simulink model "w31_v6"  (Simulink 7.9)
settings: Solver=FixedStepDiscrete  StartTime=0.0  StopTime=inf  FixedStep=0.01  RelTol=1e-3
undefined symbols (not defined in the file): DiscIntNeverNeededParam, magnitude
libraries: canmsglib x24, cansrvlib x22, simulink x12, iohwablib x5, legionoslib x3, ccpsrvlib x2, memsrvlib x1, tgttoollib x1, udssrvlib x1, wdgmlib x1
(part 1 of 5)
settings Model: Creator=jjlong  LastModifiedBy=申棋仁
settings DataIOCC: SaveOutput=off  SignalLogging=off  DSMLogging=off  SaveTime=off
settings OptimizationCC: InlineParams=on  ZeroExternalMemoryAtStartup=off  NoFixptDivByZeroProtection=on  EfficientFloat2IntCast=on  OptimizeModelRefInitCode=on  LifeSpan=1
settings DebuggingCC: ParameterOverflowMsg=none  ParameterPrecisionLossMsg=none  FrameProcessingCompatibilityMsg=error  StrictBusMsg=Warning
settings HardwareCC: ProdBitPerChar=16  ProdBitPerInt=16  ProdBitPerPointer=16  ProdLargestAtomicInteger=Integer  ProdIntDivRoundTo=Zero  ProdEndianess=LittleEndian  ProdWordSize=16  ProdHWDeviceType=Texas Instruments->C2000
settings RTWCC: SystemTargetFile=ez_ert_rtw.tlc  TemplateMakefile=ez_ert_rtw.tmf  Description=ControlKernel(tm) Rapid Prototyping  ProcessScript=ez_ert_rtw_make_rtw_hook
settings CodeAppCC: IgnoreCustomStorageClasses=off
settings STFCustomTargetCC: CodeReplacementLibrary=C89/C90 (ANSI)  CompOptLevelCompliant=on  IncludeMdlTerminateFcn=off  CombineOutputUpdateFcns=on  ERTFirstTimeCompliant=on  ERTCustomFileBanners=on  SupportNonFinite=off  SupportContinuousTime=off  SupportNonInlinedSFcns=off  GRTInterface=off  SystemTargetFile=ez_ert_rtw.tlc
settings ERTTargetCC: TargetLibSuffix=.lib  CodeReplacementLibrary=C89/C90 (ANSI)  MultiwordLength=2048  ParMdlRefBuildCompliant=off  ConcurrentExecutionCompliant=off  IncludeMdlTerminateFcn=off  SupportNonFinite=off  ModelStepFunctionPrototypeControlCompliant=off  CPPClassGenCompliant=off  GenerateASAP2=on  ExtModeMexFile=noextcomm  InlinedParameterPlacement=NonHierarchical  ERTCustomFileTemplate=example_file_process.tlc  ConvertIfToSwitch=off  SuppressUnreachableDefaultCases=off  EnableUserReplacementTypes=on
settings MATStruct: double=float64  single=float32  int32=sint32  int16=sint16  int8=sint8  uint32=uint32  uint16=uint16  uint8=uint8  boolean=boolean
settings CustomProperty: Value=on

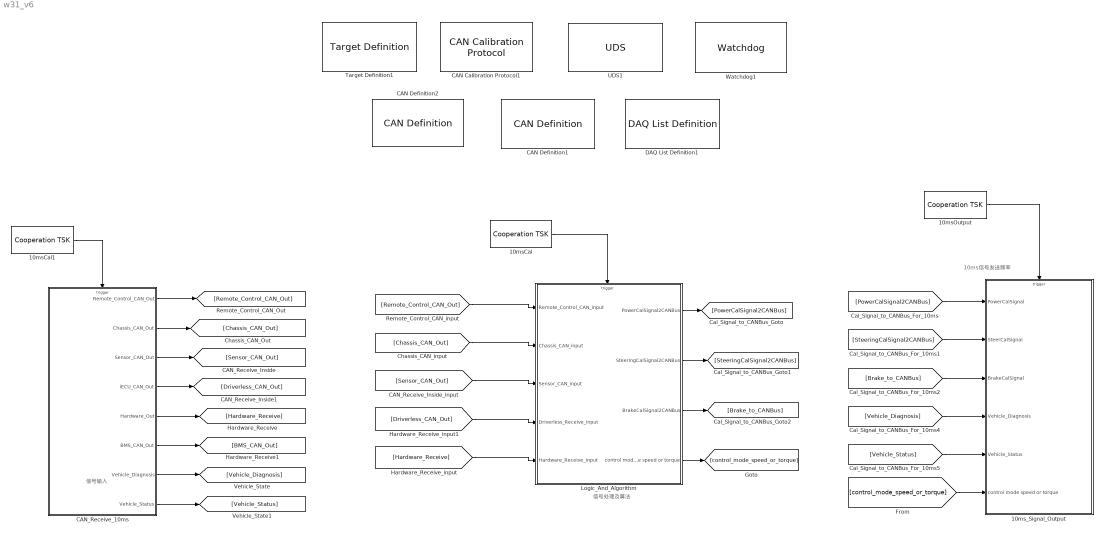
== system w31_v6 ==
  note: 信号输入
  note: 信号处理及算法
  note: 10ms信号发送频率
  10msCal : legionoslib/Cooperation TSK  taskname='task10ms1'  taskperiod=0.01  taskpriority=SCHEDCFG_DEFAULT  taskorder=1
  10msCal1 : legionoslib/Cooperation TSK  taskname='task10ms0'  taskperiod=0.01  taskpriority=SCHEDCFG_DEFAULT  taskorder=0
  10msOutput : legionoslib/Cooperation TSK  taskname='OutPut'  taskperiod=0.01  taskpriority=SCHEDCFG_DEFAULT  taskorder=2
  10ms_Signal_Output : Subsystem  TreatAsAtomicUnit=on
  CAN Calibration Protocol1 : ccpsrvlib/CAN Calibration Protocol  CCP_STATION_ID=hex2dec('1')  module=CAN2  ccp_cro_id=hex2dec('6FA')  ccp_cro_message_type=Standard (11-bit identifier)  ccp_return_id=hex2dec('6FB')  ccp_return_message_type=Standard (11-bit identifier)  ECU=V11P51_00E170701_01
      link override Receive CRO/CRO/CAN Receive: useModule=CAN2  messageType=Standard (11-bit identifier)  messageID_Numeric=1786  ECU=V11P51_00E170701_01
      link override Transmit CRM/CRM/CAN Transmit: useModule=CAN2  messageType=Standard (11-bit identifier)  messageID_Numeric=1787  ECU=V11P51_00E170701_01
  CAN Definition1 : cansrvlib/CAN Definition  useModule=CAN1  baud_rate=500  user_baud_rate=[]  ECU=V11P51_00E170701_01
  CAN Definition2 : cansrvlib/CAN Definition  useModule=CAN2  baud_rate=250  user_baud_rate=[]  ECU=V11P51_00E170701_01
  CAN_Receive_10ms : Subsystem  TreatAsAtomicUnit=on
  DAQ List Definition1 : ccpsrvlib/DAQ List Definition  list_info=[10 20;200 60]
  Logic_And_Algorithm : Subsystem  TreatAsAtomicUnit=on
  Target Definition1 : tgttoollib/Target Definition  series=Vehicle  target=V11P51_00E170701_01  cpu_clock=80  os=LGRTOS  stack_size=1024  ide=c2000_6.1.3  version=V11P310E2016123002  support_eep=on
  UDS1 : udssrvlib/UDS  module=CAN2  uds_cantx_id=hex2dec('7C9')  uds_cantx_message_type=Standard (11-bit identifier)  uds_canrx_id=hex2dec('7C1')  uds_canrx_message_type=Standard (11-bit identifier)  udstype=UDS Basic  ECU=V11P51_00E170701_01
  Watchdog1 : wdgmlib/Watchdog  mode_type=WDGIF_FAST_MODE  genr_ISR=off
  wires:
  CAN_Receive_10ms/1(Remote_Control_CAN_Out) -> [Remote_Control_CAN_Out]
  CAN_Receive_10ms/2(Chassis_CAN_Out) -> [Chassis_CAN_Out]
  CAN_Receive_10ms/3(Sensor_CAN_Out) -> [Sensor_CAN_Out]
  CAN_Receive_10ms/5(Hardware_Out) -> [Hardware_Receive]
  CAN_Receive_10ms/4(iECU_CAN_Out) -> [Driverless_CAN_Out]
  10msCal1/1 -> CAN_Receive_10ms/Trigger
  [Remote_Control_CAN_Out] -> Logic_And_Algorithm/1(Remote_Control_CAN_input)
  [Chassis_CAN_Out] -> Logic_And_Algorithm/2(Chassis_CAN_input)
  [Sensor_CAN_Out] -> Logic_And_Algorithm/3(Sensor_CAN_input)
  [Hardware_Receive] -> Logic_And_Algorithm/5(Hardware_Receive_input)
  Logic_And_Algorithm/1(PowerCalSignal2CANBus) -> [PowerCalSignal2CANBus]
  [Driverless_CAN_Out] -> Logic_And_Algorithm/4(Driverless_Receive_input)
  10msCal/1 -> Logic_And_Algorithm/Trigger
  [PowerCalSignal2CANBus] -> 10ms_Signal_Output/1(PowerCalSignal)
  10msOutput/1 -> 10ms_Signal_Output/Trigger
  Logic_And_Algorithm/2(SteeringCalSignal2CANBus) -> [SteeringCalSignal2CANBus]
  [SteeringCalSignal2CANBus] -> 10ms_Signal_Output/2(SteerCalSignal)
  Logic_And_Algorithm/3(BrakeCalSignal2CANBus) -> [Brake_to_CANBus]
  [Brake_to_CANBus] -> 10ms_Signal_Output/3(BrakeCalSignal)
  CAN_Receive_10ms/6(BMS_CAN_Out) -> [BMS_CAN_Out]
  CAN_Receive_10ms/7(Vehicle_Diagnosis) -> [Vehicle_Diagnosis]
  [Vehicle_Diagnosis] -> 10ms_Signal_Output/4(Vehicle_Diagnosis)
  CAN_Receive_10ms/8(Vehicle_Status) -> [Vehicle_Status]
  [Vehicle_Status] -> 10ms_Signal_Output/5(Vehicle_Status)
  Logic_And_Algorithm/4(control mode speed or torque) -> [control_mode_speed_or_torque]
  [control_mode_speed_or_torque] -> 10ms_Signal_Output/6(control mode speed or torque)

== system w31_v6/10ms_Signal_Output ==
  PowerCalSignal : Inport
  SteerCalSignal : Inport  Port=2
  BrakeCalSignal : Inport  Port=3
  Vehicle_Diagnosis : Inport  Port=4
  Vehicle_Status : Inport  Port=5
  control mode speed or torque : Inport  Port=6
  function : TriggerPort  TriggerType=function-call
  BrakeCAN_Out : Subsystem
  PowerCAN_Out : Subsystem
  SteerCAN_Out1 : Subsystem
  SteerCAN_Out2 : Subsystem
  Vehicle_Diagnosis_Out : Subsystem
  Vehicle_Status_Out : Subsystem
  wires:
  PowerCalSignal/1 -> PowerCAN_Out/1(PowerCalSignal), [PowerCalSignal]
  SteerCalSignal/1 -> SteerCAN_Out1/1(SteerCalSignal)
  BrakeCalSignal/1 -> BrakeCAN_Out/1(BrakeCalSignal)
  Vehicle_Diagnosis/1 -> Vehicle_Diagnosis_Out/1(Vehicle_Diagnosis)
  Vehicle_Status/1 -> Vehicle_Status_Out/1(Vehicle_Status)
  control mode speed or torque/1 -> PowerCAN_Out/2(control mode)

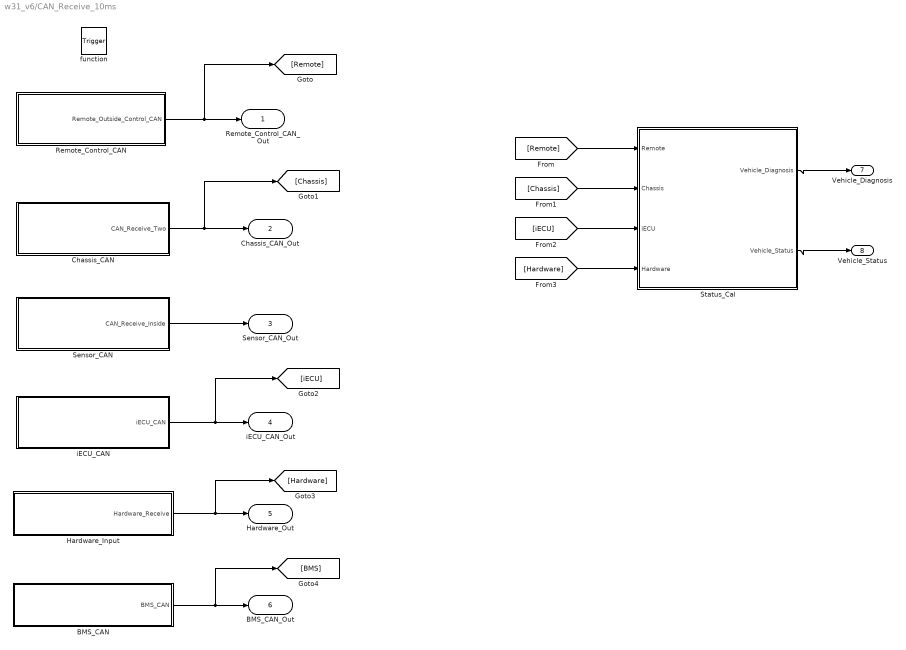
== system w31_v6/CAN_Receive_10ms ==
  function : TriggerPort  TriggerType=function-call
  BMS_CAN : Subsystem
  Chassis_CAN : Subsystem
  Hardware_Input : Subsystem
  Remote_Control_CAN : Subsystem
  Sensor_CAN : Subsystem
  Status_Cal : Subsystem
  iECU_CAN : Subsystem
  Remote_Control_CAN_Out : Outport
  Chassis_CAN_Out : Outport  Port=2
  Sensor_CAN_Out : Outport  Port=3
  iECU_CAN_Out : Outport  Port=4
  Hardware_Out : Outport  Port=5
  BMS_CAN_Out : Outport  Port=6
  Vehicle_Diagnosis : Outport  Port=7
  Vehicle_Status : Outport  Port=8
  wires:
  Remote_Control_CAN/1(Remote_Outside_Control_CAN) -> Remote_Control_CAN_Out/1, [Remote]
  Chassis_CAN/1(CAN_Receive_Two) -> Chassis_CAN_Out/1, [Chassis]
  Sensor_CAN/1(CAN_Receive_Inside) -> Sensor_CAN_Out/1
  Hardware_Input/1(Hardware_Receive) -> Hardware_Out/1, [Hardware]
  iECU_CAN/1(iECU_CAN) -> iECU_CAN_Out/1, [iECU]
  BMS_CAN/1(BMS_CAN) -> BMS_CAN_Out/1, [BMS]
  [Remote] -> Status_Cal/1(Remote)
  [Chassis] -> Status_Cal/2(Chassis)
  [iECU] -> Status_Cal/3(iECU)
  [Hardware] -> Status_Cal/4(Hardware)
  Status_Cal/1(Vehicle_Diagnosis) -> Vehicle_Diagnosis/1
  Status_Cal/2(Vehicle_Status) -> Vehicle_Status/1

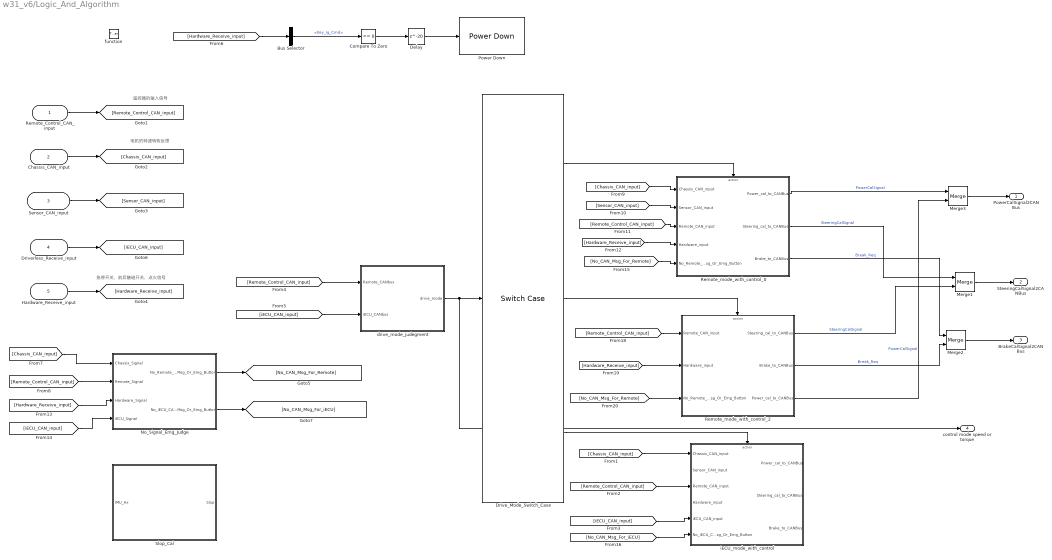
== system w31_v6/Logic_And_Algorithm ==
  note: 遥控器的输入信号
  note: 急停开关、前后触碰开关、点火信号
  note: 电机的转速转矩反馈
  Remote_Control_CAN_input : Inport
  Chassis_CAN_input : Inport  Port=2
  Sensor_CAN_input : Inport  Port=3
  Driverless_Receive_input : Inport  Port=4
  Hardware_Receive_input : Inport  Port=5
  function : TriggerPort  TriggerType=function-call
  Bus Selector : BusSelector  OutputSignals=Key_Ig_Cmd
  Compare To Zero : simulink/Logic and Bit Operations/Compare To Zero  relop===  OutDataTypeStr=boolean
  Delay : Delay  DelayLength=20
  Drive_Mode_Switch_Case : SwitchCase  CaseConditions={0,2}
  Merge1 : Merge
  Merge2 : Merge
  Merge3 : Merge
  No_Signal_Emg_Judge : Subsystem
  Power Down : memsrvlib/Power Down
  Remote_mode_with_control_0 : Subsystem  TreatAsAtomicUnit=on
  Remote_mode_with_control_2 : Subsystem  TreatAsAtomicUnit=on
  Slop_Cal : Subsystem
  drive_mode_judegment : Subsystem
  iECU_mode_with_control : Subsystem  TreatAsAtomicUnit=on
  PowerCalSignal2CANBus : Outport
  SteeringCalSignal2CANBus : Outport  Port=2
  BrakeCalSignal2CANBus : Outport  Port=3
  control mode speed or torque : Outport  Port=4
  wires:
  Remote_Control_CAN_input/1 -> [Remote_Control_CAN_input]
  Chassis_CAN_input/1 -> [Chassis_CAN_input]
  Sensor_CAN_input/1 -> [Sensor_CAN_input]
  Hardware_Receive_input/1 -> [Hardware_Receive_input]
  Driverless_Receive_input/1 -> [iECU_CAN_input]
  [Chassis_CAN_input] -> Remote_mode_with_control_0/1(Chassis_CAN_input)
  [Sensor_CAN_input] -> Remote_mode_with_control_0/2(Sensor_CAN_input)
  [Remote_Control_CAN_input] -> Remote_mode_with_control_0/3(Remote_CAN_input)
  [Hardware_Receive_input] -> Remote_mode_with_control_0/4(Hardware_input)
  Compare To Zero/1 -> Delay/1
  Delay/1 -> Power Down/1
  Bus Selector/1 -> Compare To Zero/1  "<Key_Ig_Cmd>"
  Drive_Mode_Switch_Case/1 -> Remote_mode_with_control_0/Action
  Drive_Mode_Switch_Case/3 -> iECU_mode_with_control/Action
  [Chassis_CAN_input] -> iECU_mode_with_control/1(Chassis_CAN_input)
  [Remote_Control_CAN_input] -> iECU_mode_with_control/3(Remote_CAN_input)
  [iECU_CAN_input] -> iECU_mode_with_control/5(iECU_CAN_input)
  Remote_mode_with_control_0/2(Steering_cal_to_CANBus) -> Merge1/1  "SteeringCalSignal"
  Merge1/1 -> SteeringCalSignal2CANBus/1
  drive_mode_judegment/1(drive_mode) -> Drive_Mode_Switch_Case/1, control mode speed or torque/1
  [Remote_Control_CAN_input] -> drive_mode_judegment/1(Remote_CANbus)
  [iECU_CAN_input] -> drive_mode_judegment/2(iECU_CANbus)
  [Hardware_Receive_input] -> Bus Selector/1
  [Chassis_CAN_input] -> No_Signal_Emg_Judge/1(Chassis_Signal)
  [Remote_Control_CAN_input] -> No_Signal_Emg_Judge/2(Remote_Signal)
  [Hardware_Receive_input] -> No_Signal_Emg_Judge/3(Hardware_Signal)
  [iECU_CAN_input] -> No_Signal_Emg_Judge/4(iECU_Signal)
  No_Signal_Emg_Judge/1(No_Remote_CAN_Msg_Or_Emg_Button) -> [No_CAN_Msg_For_Remote]
  No_Signal_Emg_Judge/2(No_iECU_CAN_Msg_Or_Emg_Button) -> [No_CAN_Msg_For_iECU]
  [No_CAN_Msg_For_Remote] -> Remote_mode_with_control_0/5(No_Remote_CAN_Msg_Or_Emg_Button)
  [No_CAN_Msg_For_iECU] -> iECU_mode_with_control/6(No_iECU_CAN_Msg_Or_Emg_Button)
  [Hardware_Receive_input] -> Remote_mode_with_control_2/2(Hardware_input)
  [No_CAN_Msg_For_Remote] -> Remote_mode_with_control_2/3(No_Remote_CAN_Msg_Or_Emg_Button)
  [Remote_Control_CAN_input] -> Remote_mode_with_control_2/1(Remote_CAN_input)
  Drive_Mode_Switch_Case/2 -> Remote_mode_with_control_2/Action
  Merge2/1 -> BrakeCalSignal2CANBus/1
  Remote_mode_with_control_0/3(Brake_to_CANBus) -> Merge2/1  "Break_Req"
  Remote_mode_with_control_2/2(Brake_to_CANBus) -> Merge2/2  "Break_Req"
  Remote_mode_with_control_2/1(Steering_cal_to_CANBus) -> Merge1/2  "SteeringCalSignal"
  Remote_mode_with_control_0/1(Power_cal_to_CANBus) -> Merge3/1  "PowerCalSignal"
  Remote_mode_with_control_2/3(Power_cal_to_CANBus) -> Merge3/2  "PowerCalSignal"
  Merge3/1 -> PowerCalSignal2CANBus/1

== system w31_v6/10ms_Signal_Output/BrakeCAN_Out ==
  BrakeCalSignal : Inport
  1-D Lookup Table : Lookup_n-D  NumberOfTableDimensions=1  BreakpointsForDimension1=[0,0.5,1,1.5,2,2.5,3,3.5,4]  Table=[0,0.20155,0.33592,0.44961,0.70801,0.94574,1.4109,2.4548,4]  RndMeth=Simplest  InputSameDT=on
  Bus Selector : BusSelector  OutputSignals=Break_Req,Remote_EPB_Req
  CAN Pack1 : canmsglib/CAN Pack  CANdbFile=E:\matlab_ws\2012_Matlab_Vcu\w_serial\w3\w31\子系统\EPB\dbc\EPB_test.dbc  MsgList=VCU_EPB_Request_310  MsgName=VCU_EPB_Request_310  MsgIDType=Standard (11-bit identifier)  MsgIdentifier=784  MsgLength=8  SignalInfo=FlagVCU_EPB_Request$2$1$1$2$1$0$1$0$0$1$#VCU_EPB_Parking_Request$0$2$1$2$1$0$1$0$0$3$#  NSignals=2  StartBits=str2num('[int32(2);int32(0)]')  SignalSizes=str2num('[int32(1);int32(2)]')  ByteOrders=str2num('[int32(1);int32(1)]')  DataTypes=str2num('[int32(2);int32(2)]')  MultiplexTypes=str2num('[int32(1);int32(1)]')  MultiplexValues=str2num('[double(0);double(0)]')  Factors=str2num('[double(1);double(1)]')  Offsets=str2num('[double(0);double(0)]')  Minimums=str2num('[double(0);double(0)]')  Maximums=str2num('[double(1);double(3)]')  Remote=off
      settings: DataFormat=CANdb specified signals
  CAN Pack2 : canmsglib/CAN Pack  CANdbFile=E:\matlab_ws\2012_Matlab_Vcu\w_serial\w3\w32\dbc\w32_CAN1_500kbs_0319_v6.dbc  MsgList=VCU_IBCF_Request  MsgName=VCU_IBCF_Request  MsgIDType=Standard (11-bit identifier)  MsgIdentifier=340  MsgLength=7  SignalInfo=Reserved_1$0$17$1$1$1$0$1$0$-Inf$Inf$#Reserved_2$18$7$1$1$1$0$1$0$0$8$#VCU_Break_Pressure_Request$40$16$1$2$1$0$1.000000e-02$0$0$8$#VCU_Break_Request_Flag$17$1$1$2$1$0$1$0$0$2$#  NSignals=4  StartBits=str2num('[int32(0);int32(18);int32(40);int32(17)]')  SignalSizes=str2num('[int32(17);int32(7);int32(16);int32(1)]')  ByteOrders=str2num('[int32(1);int32(1);int32(1);int32(1)]')  DataTypes=str2num('[int32(1);int32(1);int32(2);int32(2)]')  MultiplexTypes=str2num('[int32(1);int32(1);int32(1);int32(1)]')  MultiplexValues=str2num('[double(0);double(0);double(0);double(0)]')  Factors=str2num('[double(1);double(1);double(1.000000e-02);double(1)]')  Offsets=str2num('[double(0);double(0);double(0);double(0)]')  Minimums=str2num('[double(-Inf);double(0);double(0);double(0)]')  Maximums=str2num('[double(Inf);double(8);double(8);double(2)]')  Remote=off
      settings: DataFormat=CANdb specified signals
  CAN Transmit1 : cansrvlib/CAN Transmit  useModule=CAN1  messageID=hex2dec('154')  messageType=Standard (11-bit identifier)  msg_priority=255  messageID_Numeric=340  ECU=V11P51_00E170701_01
  CAN Transmit2 : cansrvlib/CAN Transmit  useModule=CAN1  messageID=hex2dec('310')  messageType=Standard (11-bit identifier)  msg_priority=255  messageID_Numeric=784  ECU=V11P51_00E170701_01
  Constant : Constant  OutDataTypeStr=uint8  SampleTime=-1
  Constant1 : Constant  Value=0  OutDataTypeStr=uint8  SampleTime=-1
  wires:
  CAN Pack2/1 -> CAN Transmit1/1
  Constant/1 -> CAN Pack2/4
  1-D Lookup Table/1 -> CAN Pack2/3
  Bus Selector/1 -> 1-D Lookup Table/1  "<Break_Req>"
  CAN Pack1/1 -> CAN Transmit2/1
  Constant1/1 -> CAN Pack1/1
  Bus Selector/2 -> CAN Pack1/2  "<Remote_EPB_Req>"
  BrakeCalSignal/1 -> Bus Selector/1

== system w31_v6/10ms_Signal_Output/PowerCAN_Out ==
  PowerCalSignal : Inport
  control mode : Inport  Port=2
  Bus Selector1 : BusSelector  OutputSignals=Power_FL,Power_FR,Power_RL,Power_RR
  CAN Pack1 : canmsglib/CAN Pack  CANdbFile=D:\W31_workspace\w31_CAN1_500kbs_0618_v5.1.dbc  MsgList=VCU_MCURL_Request_1  MsgName=VCU_MCURL_Request_1  MsgIDType=Standard (11-bit identifier)  MsgIdentifier=384  MsgLength=8  SignalInfo=RL_DriveMode$1$2$1$2$1$0$1$0$0$3$#RL_Reserved_1$3$5$1$2$1$0$1$0$0$31$#RL_Reserved_2$40$24$1$2$1$0$1$0$0$255$#RL_Speed_Req$24$16$1$2$1$0$1$-7000$-7000$7000$#RL_Torque_Req$8$16$1$2$1$0$1.000000e-01$-1000$-1000$1000$#RL_VCU_Motor_Request_Valid$0$1$1$2$1$0$1$0$0$1$#  NSignals=6  StartBits=str2num('[int32(1);int32(3);int32(40);int32(24);int32(8);int32(0)]')  SignalSizes=str2num('[int32(2);int32(5);int32(24);int32(16);int32(16);int32(1)]')  ByteOrders=str2num('[int32(1);int32(1);int32(1);int32(1);int32(1);int32(1)]')  DataTypes=str2num('[int32(2);int32(2);int32(2);int32(2);int32(2);int32(2)]')  MultiplexTypes=str2num('[int32(1);int32(1);int32(1);int32(1);int32(1);int32(1)]')  MultiplexValues=str2num('[double(0);double(0);double(0);double(0);double(0);double(0)]')  Factors=str2num('[double(1);double(1);double(1);double(1);double(1.000000e-01);double(1)]')  Offsets=str2num('[double(0);double(0);double(0);double(-7000);double(-1000);double(0)]')  Minimums=str2num('[double(0);double(0);double(0);double(-7000);double(-1000);double(0)]')  Maximums=str2num('[double(3);double(31);double(255);double(7000);double(1000);double(1)]')  Remote=off
      settings: DataFormat=CANdb specified signals
  CAN Pack2 : canmsglib/CAN Pack  CANdbFile=D:\W31_workspace\w31_CAN1_500kbs_0618_v5.1.dbc  MsgList=VCU_MCURR_Request_1  MsgName=VCU_MCURR_Request_1  MsgIDType=Standard (11-bit identifier)  MsgIdentifier=400  MsgLength=8  SignalInfo=RR_DriveMode$1$2$1$2$1$0$1$0$0$3$#RR_Reserved_1$3$5$1$2$1$0$1$0$0$31$#RR_Reserved_2$40$24$1$2$1$0$1$0$0$255$#RR_Speed_Req$24$16$1$2$1$0$1$-7000$-7000$7000$#RR_Torque_Req$8$16$1$2$1$0$1.000000e-01$-1000$-1000$1000$#RR_VCU_Motor_Request_Valid$0$1$1$2$1$0$1$0$0$1$#  NSignals=6  StartBits=str2num('[int32(1);int32(3);int32(40);int32(24);int32(8);int32(0)]')  SignalSizes=str2num('[int32(2);int32(5);int32(24);int32(16);int32(16);int32(1)]')  ByteOrders=str2num('[int32(1);int32(1);int32(1);int32(1);int32(1);int32(1)]')  DataTypes=str2num('[int32(2);int32(2);int32(2);int32(2);int32(2);int32(2)]')  MultiplexTypes=str2num('[int32(1);int32(1);int32(1);int32(1);int32(1);int32(1)]')  MultiplexValues=str2num('[double(0);double(0);double(0);double(0);double(0);double(0)]')  Factors=str2num('[double(1);double(1);double(1);double(1);double(1.000000e-01);double(1)]')  Offsets=str2num('[double(0);double(0);double(0);double(-7000);double(-1000);double(0)]')  Minimums=str2num('[double(0);double(0);double(0);double(-7000);double(-1000);double(0)]')  Maximums=str2num('[double(3);double(31);double(255);double(7000);double(1000);double(1)]')  Remote=off
      settings: DataFormat=CANdb specified signals
  CAN Pack3 : canmsglib/CAN Pack  CANdbFile=D:\W31_workspace\w31_CAN1_500kbs_0618_v5.1.dbc  MsgList=VCU_MCUFL_Request_1  MsgName=VCU_MCUFL_Request_1  MsgIDType=Standard (11-bit identifier)  MsgIdentifier=352  MsgLength=8  SignalInfo=FL_DriveMode$1$2$1$2$1$0$1$0$0$3$#FL_Reserved_1$3$5$1$2$1$0$1$0$0$31$#FL_Reserved_2$40$24$1$2$1$0$1$0$0$255$#FL_Speed_Req$24$16$1$2$1$0$1$-7000$-7000$7000$#FL_Torque_Req$8$16$1$2$1$0$1.000000e-01$-1000$-1000$1000$#FL_VCU_Motor_Request_Valid$0$1$1$2$1$0$1$0$0$1$#  NSignals=6  StartBits=str2num('[int32(1);int32(3);int32(40);int32(24);int32(8);int32(0)]')  SignalSizes=str2num('[int32(2);int32(5);int32(24);int32(16);int32(16);int32(1)]')  ByteOrders=str2num('[int32(1);int32(1);int32(1);int32(1);int32(1);int32(1)]')  DataTypes=str2num('[int32(2);int32(2);int32(2);int32(2);int32(2);int32(2)]')  MultiplexTypes=str2num('[int32(1);int32(1);int32(1);int32(1);int32(1);int32(1)]')  MultiplexValues=str2num('[double(0);double(0);double(0);double(0);double(0);double(0)]')  Factors=str2num('[double(1);double(1);double(1);double(1);double(1.000000e-01);double(1)]')  Offsets=str2num('[double(0);double(0);double(0);double(-7000);double(-1000);double(0)]')  Minimums=str2num('[double(0);double(0);double(0);double(-7000);double(-1000);double(0)]')  Maximums=str2num('[double(3);double(31);double(255);double(7000);double(1000);double(1)]')  Remote=off
      settings: DataFormat=CANdb specified signals
  CAN Pack4 : canmsglib/CAN Pack  CANdbFile=D:\W31_workspace\w31_CAN1_500kbs_0618_v5.1.dbc  MsgList=VCU_MCUFR_Request_1  MsgName=VCU_MCUFR_Request_1  MsgIDType=Standard (11-bit identifier)  MsgIdentifier=368  MsgLength=8  SignalInfo=FR_DriveMode$1$2$1$2$1$0$1$0$0$3$#FR_Reserved_1$3$5$1$2$1$0$1$0$0$31$#FR_Reserved_2$40$24$1$2$1$0$1$0$0$255$#FR_Speed_Req$24$16$1$2$1$0$1$-7000$-7000$7000$#FR_Torque_Req$8$16$1$2$1$0$1.000000e-01$-1000$-1000$1000$#FR_VCU_Motor_Request_Valid$0$1$1$2$1$0$1$0$0$1$#  NSignals=6  StartBits=str2num('[int32(1);int32(3);int32(40);int32(24);int32(8);int32(0)]')  SignalSizes=str2num('[int32(2);int32(5);int32(24);int32(16);int32(16);int32(1)]')  ByteOrders=str2num('[int32(1);int32(1);int32(1);int32(1);int32(1);int32(1)]')  DataTypes=str2num('[int32(2);int32(2);int32(2);int32(2);int32(2);int32(2)]')  MultiplexTypes=str2num('[int32(1);int32(1);int32(1);int32(1);int32(1);int32(1)]')  MultiplexValues=str2num('[double(0);double(0);double(0);double(0);double(0);double(0)]')  Factors=str2num('[double(1);double(1);double(1);double(1);double(1.000000e-01);double(1)]')  Offsets=str2num('[double(0);double(0);double(0);double(-7000);double(-1000);double(0)]')  Minimums=str2num('[double(0);double(0);double(0);double(-7000);double(-1000);double(0)]')  Maximums=str2num('[double(3);double(31);double(255);double(7000);double(1000);double(1)]')  Remote=off
      settings: DataFormat=CANdb specified signals
  CAN Transmit1 : cansrvlib/CAN Transmit  useModule=CAN1  messageID=hex2dec('180')  messageType=Standard (11-bit identifier)  msg_priority=255  messageID_Numeric=384  ECU=V11P51_00E170701_01
  CAN Transmit2 : cansrvlib/CAN Transmit  useModule=CAN1  messageID=hex2dec('190')  messageType=Standard (11-bit identifier)  msg_priority=255  messageID_Numeric=400  ECU=V11P51_00E170701_01
  CAN Transmit3 : cansrvlib/CAN Transmit  useModule=CAN1  messageID=hex2dec('160')  messageType=Standard (11-bit identifier)  msg_priority=255  messageID_Numeric=352  ECU=V11P51_00E170701_01
  CAN Transmit4 : cansrvlib/CAN Transmit  useModule=CAN1  messageID=hex2dec('170')  messageType=Standard (11-bit identifier)  msg_priority=255  messageID_Numeric=368  ECU=V11P51_00E170701_01
  Constant : Constant  Value=3
  Constant1 : Constant  Value=2
  Constant2 : Constant
  Gain : Gain
  Gain1 : Gain  Gain=-1
  Gain2 : Gain
  Gain3 : Gain  Gain=-1
  Saturation{,1..3} (4 alike) : Saturate  UpperLimit=500  LowerLimit=-500
  Switch : Switch  Criteria=u2 ~= 0
  wires:
  PowerCalSignal/1 -> Bus Selector1/1
  control mode/1 -> Switch/2
  Constant1/1 -> Switch/1
  Constant/1 -> Switch/3
  Bus Selector1/1 -> Gain/1  "<Power_FL>"
  Bus Selector1/2 -> Gain1/1  "<Power_FR>"
  Bus Selector1/3 -> Gain2/1  "<Power_RL>"
  Bus Selector1/4 -> Gain3/1  "<Power_RR>"
  Switch/1 -> CAN Pack3/1, CAN Pack4/1, CAN Pack1/1, CAN Pack2/1
  Constant2/1 -> CAN Pack3/6, CAN Pack4/6, CAN Pack1/6, CAN Pack2/6
  Gain/1 -> CAN Pack3/5, Saturation/1
  Gain1/1 -> CAN Pack4/5, Saturation1/1
  Gain2/1 -> CAN Pack1/5, Saturation2/1
  Gain3/1 -> CAN Pack2/5, Saturation3/1
  CAN Pack3/1 -> CAN Transmit3/1
  CAN Pack4/1 -> CAN Transmit4/1
  CAN Pack1/1 -> CAN Transmit1/1
  CAN Pack2/1 -> CAN Transmit2/1
  Saturation/1 -> CAN Pack3/4
  Saturation1/1 -> CAN Pack4/4
  Saturation2/1 -> CAN Pack1/4
  Saturation3/1 -> CAN Pack2/4

== system w31_v6/10ms_Signal_Output/SteerCAN_Out1 ==
  SteerCalSignal : Inport
  Bus Selector1 : BusSelector  OutputSignals=F_Steering_Angle,R_Steering_Angle
  F : Subsystem
  R : Subsystem
  wires:
  SteerCalSignal/1 -> Bus Selector1/1
  Bus Selector1/1 -> F/1(Command_Angle)  "<F_Steering_Angle>"
  Bus Selector1/2 -> R/1(Command_Angle)  "<R_Steering_Angle>"

== system w31_v6/10ms_Signal_Output/SteerCAN_Out2 ==
  DO5 : iohwablib/DO  text_resource=LSO6  use_diag=off  ECU=V11P51_00E170701_01
  Status_Light : Constant  OutDataTypeStr=Inherit: Inherit via back propagation  SampleTime=-1
  wires:
  Status_Light/1 -> DO5/1

== system w31_v6/10ms_Signal_Output/Vehicle_Diagnosis_Out ==
  Vehicle_Diagnosis : Inport
  Bus Selector : BusSelector  OutputSignals=Chassis_Status.DBSF_Status_NoRxMsg,Hardware_Status.Eme_Stop_Cmd,Chassis_Status.FL_Motor_Status_NoRxMsg,Chassis_Status.FR_Motor_Status_NoRxMsg,Chassis_Status.EPSF_Status_NoRxMsg,Chassis_Status.RL_Motor_Status_NoRxMsg,Chassis_Status.RR_Motor_Status_NoRxMsg,Chassis_Status.EPSR_Status_NoRxMsg,Remote_Status.Remote_Status,iECU_Status.iECU_Status
  CAN Pack2 : canmsglib/CAN Pack  CANdbFile=E:\matlab_ws\2012_Matlab_Vcu\w_serial\w3\w32\dbc\w32_CAN1_500kbs_0327_v9.dbc  MsgList=VCU_Vehicle_Diagnosis  MsgName=VCU_Vehicle_Diagnosis  MsgIDType=Standard (11-bit identifier)  MsgIdentifier=769  MsgLength=8  SignalInfo=BMS_State$6$1$1$2$1$0$1$0$0$1$#DBSF_State$7$1$1$2$1$0$1$0$0$1$#DBSR_State$8$1$1$2$1$0$1$0$0$1$#Emergency_Button_State$0$1$1$2$1$0$1$0$0$1$#FLMotor_State$2$1$1$2$1$0$1$0$0$1$#FRMotor_State$1$1$1$2$1$0$1$0$0$1$#FSteering_State$10$1$1$2$1$0$1$0$0$1$#RLMotor_State$4$1$1$2$1$0$1$0$0$1$#RRMotor_State$3$1$1$2$1$0$1$0$0$1$#RSteering_State$11$1$1$2$1$0$1$0$0$1$#Remote_State$5$1$1$2$1$0$1$0$0$1$#iECU_State$12$1$1$2$1$0$1$0$0$1$#  NSignals=12  StartBits=str2num('[int32(6);int32(7);int32(8);int32(0);int32(2);int32(1);int32(10);int32(4);int32(3);int32(11);int32(5);int32(12)]')  SignalSizes=str2num('[int32(1);int32(1);int32(1);int32(1);int32(1);int32(1);int32(1);int32(1);int32(1);int32(1);int32(1);int32(1)]')  ByteOrders=str2num('[int32(1);int32(1);int32(1);int32(1);int32(1);int32(1);int32(1);int32(1);int32(1);int32(1);int32(1);int32(1)]')  DataTypes=str2num('[int32(2);int32(2);int32(2);int32(2);int32(2);int32(2);int32(2);int32(2);int32(2);int32(2);int32(2);int32(2)]')  MultiplexTypes=str2num('[int32(1);int32(1);int32(1);int32(1);int32(1);int32(1);int32(1);int32(1);int32(1);int32(1);int32(1);int32(1)]')  MultiplexValues=str2num('[double(0);double(0);double(0);double(0);double(0);double(0);double(0);double(0);double(0);double(0);double(0);double(0)]')  Factors=str2num('[double(1);double(1);double(1);double(1);double(1);double(1);double(1);double(1);double(1);double(1);double(1);double(1)]')  Offsets=str2num('[double(0);double(0);double(0);double(0);double(0);double(0);double(0);double(0);double(0);double(0);double(0);double(0)]')  Minimums=str2num('[double(0);double(0);double(0);double(0);double(0);double(0);double(0);double(0);double(0);double(0);double(0);double(0)]')  Maximums=str2num('[double(1);double(1);double(1);double(1);double(1);double(1);double(1);double(1);double(1);double(1);double(1);double(1)]')  Remote=off
      settings: DataFormat=CANdb specified signals
  CAN Transmit1 : cansrvlib/CAN Transmit  useModule=CAN1  messageID=hex2dec('301')  messageType=Standard (11-bit identifier)  msg_priority=255  messageID_Numeric=769  ECU=V11P51_00E170701_01
  wires:
  Vehicle_Diagnosis/1 -> Bus Selector/1
  CAN Pack2/1 -> CAN Transmit1/1
  Bus Selector/1 -> CAN Pack2/2  "<DBSF_Status_NoRxMsg>"
  Bus Selector/2 -> CAN Pack2/4  "<Eme_Stop_Cmd>"
  Bus Selector/3 -> CAN Pack2/5  "<FL_Motor_Status_NoRxMsg>"
  Bus Selector/4 -> CAN Pack2/6  "<FR_Motor_Status_NoRxMsg>"
  Bus Selector/5 -> CAN Pack2/7  "<EPSF_Status_NoRxMsg>"
  Bus Selector/6 -> CAN Pack2/8  "<RL_Motor_Status_NoRxMsg>"
  Bus Selector/7 -> CAN Pack2/9  "<RR_Motor_Status_NoRxMsg>"
  Bus Selector/8 -> CAN Pack2/10  "<EPSR_Status_NoRxMsg>"
  Bus Selector/9 -> CAN Pack2/11  "<Remote_Status>"
  Bus Selector/10 -> CAN Pack2/12  "<iECU_Status>"

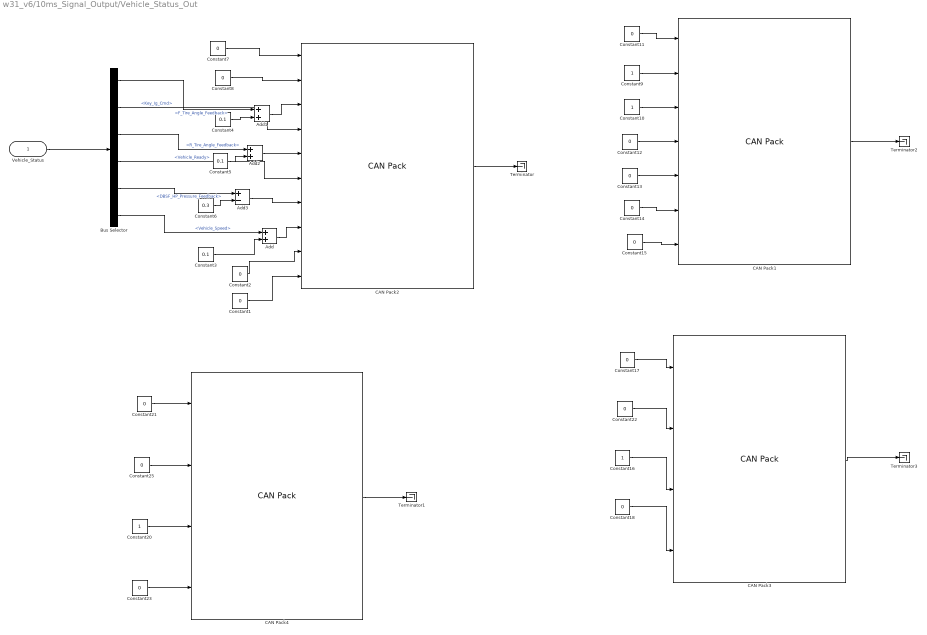
== system w31_v6/10ms_Signal_Output/Vehicle_Status_Out ==
  Vehicle_Status : Inport
  Add : Sum
  Add1 : Sum
  Add2 : Sum
  Add3 : Sum  Inputs=+-
  Bus Selector : BusSelector  OutputSignals=F_Tire_Angle_Feedback,Key_Ig_Cmd,R_Tire_Angle_Feedback,Vehicle_Ready,DBSF_HP_Pressure_Feedback,Vehicle_Speed
  CAN Pack1 : canmsglib/CAN Pack  CANdbFile=E:\matlab_ws\2012_Matlab_Vcu\w_serial\w3\w31\子系统\EPB\dbc\EPB_test.dbc  MsgList=Vehicle_Status_303  MsgName=Vehicle_Status_303  MsgIDType=Standard (11-bit identifier)  MsgIdentifier=771  MsgLength=8  SignalInfo=AccPedal$8$8$1$2$1$0$1$0$0$100$#BrakePedalStatus$3$1$1$2$1$0$1$0$0$1$#IgnitionStatus$2$1$1$2$1$0$1$0$0$1$#ShiftGear$0$2$1$2$1$0$1$0$0$3$#Vehicle_Brake_Pressure$24$8$1$2$1$0$1.000000e-01$0$0$8$#Vehicle_Speed$16$8$1$2$1$0$1$-80$-80$80$#Vehicle_Torque$32$12$1$2$1$0$1$-1000$-1000$1000$#  NSignals=7  StartBits=str2num('[int32(8);int32(3);int32(2);int32(0);int32(24);int32(16);int32(32)]')  SignalSizes=str2num('[int32(8);int32(1);int32(1);int32(2);int32(8);int32(8);int32(12)]')  ByteOrders=str2num('[int32(1);int32(1);int32(1);int32(1);int32(1);int32(1);int32(1)]')  DataTypes=str2num('[int32(2);int32(2);int32(2);int32(2);int32(2);int32(2);int32(2)]')  MultiplexTypes=str2num('[int32(1);int32(1);int32(1);int32(1);int32(1);int32(1);int32(1)]')  MultiplexValues=str2num('[double(0);double(0);double(0);double(0);double(0);double(0);double(0)]')  Factors=str2num('[double(1);double(1);double(1);double(1);double(1.000000e-01);double(1);double(1)]')  Offsets=str2num('[double(0);double(0);double(0);double(0);double(0);double(-80);double(-1000)]')  Minimums=str2num('[double(0);double(0);double(0);double(0);double(0);double(-80);double(-1000)]')  Maximums=str2num('[double(100);double(1);double(1);double(3);double(8);double(80);double(1000)]')  Remote=off
      settings: DataFormat=CANdb specified signals
  CAN Pack2 : canmsglib/CAN Pack  CANdbFile=C:\Users\Mr Sun\Desktop\SQ_WS\W31\w31_CAN1_500kbs_0605_v4.2.dbc  MsgList=VCU_Vehicle_Status  MsgName=VCU_Vehicle_Status  MsgIDType=Standard (11-bit identifier)  MsgIdentifier=771  MsgLength=8  SignalInfo=BMS_Status$2$1$1$2$1$0$1$0$0$3$#EPB_Status$3$2$1$2$1$0$1$0$0$3$#F_Tire_Angle$36$10$1$2$1$0$1.000000e-01$-30$-30$30$#IgnitionStatus$1$1$1$2$1$0$1$0$0$1$#R_Tire_Angle$46$10$1$2$1$0$1.000000e-01$-30$-30$30$#VCU_Ready_Flag$0$1$1$2$1$0$1$0$0$1$#Vehicle_Brake_Pressure$28$8$1$2$1$0$1.000000e-01$0$0$8$#Vehicle_Speed$16$12$1$2$1$0$1.000000e-01$-80$-80$80$#Vehicle_Status_Reserved$56$8$1$2$1$0$1$0$0$255$#Vehicle_Status_Reserved1$5$11$1$2$1$0$1$0$0$8191$#  NSignals=10  StartBits=str2num('[int32(2);int32(3);int32(36);int32(1);int32(46);int32(0);int32(28);int32(16);int32(56);int32(5)]')  SignalSizes=str2num('[int32(1);int32(2);int32(10);int32(1);int32(10);int32(1);int32(8);int32(12);int32(8);int32(11)]')  ByteOrders=str2num('[int32(1);int32(1);int32(1);int32(1);int32(1);int32(1);int32(1);int32(1);int32(1);int32(1)]')  DataTypes=str2num('[int32(2);int32(2);int32(2);int32(2);int32(2);int32(2);int32(2);int32(2);int32(2);int32(2)]')  MultiplexTypes=str2num('[int32(1);int32(1);int32(1);int32(1);int32(1);int32(1);int32(1);int32(1);int32(1);int32(1)]')  MultiplexValues=str2num('[double(0);double(0);double(0);double(0);double(0);double(0);double(0);double(0);double(0);double(0)]')  Factors=str2num('[double(1);double(1);double(1.000000e-01);double(1);double(1.000000e-01);double(1);double(1.000000e-01);double(1.000000e-01);double(1);double(1)]')  Offsets=str2num('[double(0);double(0);double(-30);double(0);double(-30);double(0);double(0);double(-80);double(0);double(0)]')  Minimums=str2num('[double(0);double(0);double(-30);double(0);double(-30);double(0);double(0);double(-80);double(0);double(0)]')  Maximums=str2num('[double(3);double(3);double(30);double(1);double(30);double(1);double(8);double(80);double(255);double(8191)]')  Remote=off
      settings: DataFormat=CANdb specified signals
  CAN Pack3 : canmsglib/CAN Pack  CANdbFile=E:\matlab_ws\2012_Matlab_Vcu\w_serial\w3\w31\子系统\EPB\dbc\EPB_test.dbc  MsgList=Motor_Diagnosis_301  MsgName=Motor_Diagnosis_301  MsgIDType=Standard (11-bit identifier)  MsgIdentifier=769  MsgLength=8  SignalInfo=FL_Motor_Error$1$1$1$2$1$0$1$0$0$1$#FR_Motor_Error$0$1$1$2$1$0$1$0$0$1$#RL_Motor_Error$3$1$1$2$1$0$1$0$0$1$#RR_Motor_Error$2$1$1$2$1$0$1$0$0$1$#  NSignals=4  StartBits=str2num('[int32(1);int32(0);int32(3);int32(2)]')  SignalSizes=str2num('[int32(1);int32(1);int32(1);int32(1)]')  ByteOrders=str2num('[int32(1);int32(1);int32(1);int32(1)]')  DataTypes=str2num('[int32(2);int32(2);int32(2);int32(2)]')  MultiplexTypes=str2num('[int32(1);int32(1);int32(1);int32(1)]')  MultiplexValues=str2num('[double(0);double(0);double(0);double(0)]')  Factors=str2num('[double(1);double(1);double(1);double(1)]')  Offsets=str2num('[double(0);double(0);double(0);double(0)]')  Minimums=str2num('[double(0);double(0);double(0);double(0)]')  Maximums=str2num('[double(1);double(1);double(1);double(1)]')  Remote=off
      settings: DataFormat=manually specified signals
  CAN Pack4 : canmsglib/CAN Pack  CANdbFile=E:\matlab_ws\2012_Matlab_Vcu\w_serial\w3\w31\子系统\EPB\dbc\EPB_test.dbc  MsgList=Motor_Speed_334  MsgName=Motor_Speed_334  MsgIDType=Standard (11-bit identifier)  MsgIdentifier=820  MsgLength=8  SignalInfo=Motor_Speed_of_FLW$0$8$1$2$1$0$1$-80$-80$175$#Motor_Speed_of_FRW$8$8$1$2$1$0$1$-80$-80$175$#Motor_Speed_of_RLW$16$8$1$2$1$0$1$-80$-80$175$#Motor_Speed_of_RRW$24$8$1$2$1$0$1$-80$-80$175$#  NSignals=4  StartBits=str2num('[int32(0);int32(8);int32(16);int32(24)]')  SignalSizes=str2num('[int32(8);int32(8);int32(8);int32(8)]')  ByteOrders=str2num('[int32(1);int32(1);int32(1);int32(1)]')  DataTypes=str2num('[int32(2);int32(2);int32(2);int32(2)]')  MultiplexTypes=str2num('[int32(1);int32(1);int32(1);int32(1)]')  MultiplexValues=str2num('[double(0);double(0);double(0);double(0)]')  Factors=str2num('[double(1);double(1);double(1);double(1)]')  Offsets=str2num('[double(-80);double(-80);double(-80);double(-80)]')  Minimums=str2num('[double(-80);double(-80);double(-80);double(-80)]')  Maximums=str2num('[double(175);double(175);double(175);double(175)]')  Remote=off
      settings: DataFormat=CANdb specified signals
  Constant1 : Constant  Value=0
  Constant10 : Constant  SampleTime=-1
  Constant{7..8,11..15,17..18,21..23,25} (13 alike) : Constant  Value=0  SampleTime=-1
  Constant16 : Constant  OutDataTypeStr=Inherit: Inherit via back propagation  SampleTime=-1
  Constant2 : Constant  Value=0
  Constant20 : Constant  SampleTime=-1
  Constant3 : Constant  Value=0.1
  Constant4 : Constant  Value=0.1
  Constant5 : Constant  Value=0.1
  Constant6 : Constant  Value=0.3
  Constant9 : Constant  SampleTime=-1
  Terminator{,1..3} (4 alike) : Terminator
  wires:
  Vehicle_Status/1 -> Bus Selector/1
  Bus Selector/2 -> CAN Pack2/4  "<Key_Ig_Cmd>"
  Bus Selector/4 -> CAN Pack2/6  "<Vehicle_Ready>"
  Bus Selector/6 -> Add/1  "<Vehicle_Speed>"
  Constant2/1 -> CAN Pack2/9
  Constant3/1 -> Add/2
  Add/1 -> CAN Pack2/8
  Bus Selector/1 -> Add1/1  "<F_Tire_Angle_Feedback>"
  Constant4/1 -> Add1/2
  Add1/1 -> CAN Pack2/3
  Bus Selector/3 -> Add2/1  "<R_Tire_Angle_Feedback>"
  Constant5/1 -> Add2/2
  Add2/1 -> CAN Pack2/5
  Constant6/1 -> Add3/2
  Add3/1 -> CAN Pack2/7
  Constant7/1 -> CAN Pack2/1
  Constant8/1 -> CAN Pack2/2
  Bus Selector/5 -> Add3/1  "<DBSF_HP_Pressure_Feedback>"
  CAN Pack2/1 -> Terminator/1
  CAN Pack1/1 -> Terminator2/1
  Constant9/1 -> CAN Pack1/2
  Constant10/1 -> CAN Pack1/3
  Constant11/1 -> CAN Pack1/1
  Constant12/1 -> CAN Pack1/4
  Constant13/1 -> CAN Pack1/5
  Constant14/1 -> CAN Pack1/6
  Constant15/1 -> CAN Pack1/7
  CAN Pack3/1 -> Terminator3/1
  Constant22/1 -> CAN Pack3/2
  Constant16/1 -> CAN Pack3/3
  Constant17/1 -> CAN Pack3/1
  Constant18/1 -> CAN Pack3/4
  CAN Pack4/1 -> Terminator1/1
  Constant25/1 -> CAN Pack4/2
  Constant20/1 -> CAN Pack4/3
  Constant21/1 -> CAN Pack4/1
  Constant23/1 -> CAN Pack4/4
  Constant1/1 -> CAN Pack2/10

== system w31_v6/CAN_Receive_10ms/BMS_CAN ==
  note: time
  note: 1代表主继电器闭合，0代表不吸合
  BMS : Subsystem
  Bus Creator1 : BusCreator
  remote_shake_CAN Receive1 : cansrvlib/CAN Receive  useModule=CAN2  messageID=hex2dec('18FF28F4')  messageType=Extended (29-bit identifier)  t=-1  dataType=CAN_MESSAGE_TYPE  msg_priority=255  messageID_Numeric=419375348  ECU=V11P51_00E170701_01
  shake_situation1 : Subsystem
  t10 : Constant  Value=100  OutDataTypeStr=single  SampleTime=-1
  BMS_CAN : Outport
  wires:
  remote_shake_CAN Receive1/1 -> BMS/Trigger
  remote_shake_CAN Receive1/2 -> BMS/1(msg)
  BMS/4(BMS_Stutas) -> shake_situation1/1(RxMsgCnt)
  t10/1 -> shake_situation1/2(NoRxMsgCntMax)
  Bus Creator1/1 -> BMS_CAN/1
  BMS/1(BatteryFaultGrade) -> Bus Creator1/1  "BatteryFaultGrade"
  BMS/2(DischargeRelayStatus) -> Bus Creator1/2  "DischargeRelayStatus"
  shake_situation1/1(NoRxMsgComfirm) -> Bus Creator1/4  "BMS_Status"
  BMS/3(BMS_Loss_of_Capacity) -> Bus Creator1/3  "BMS_Loss_of_Capacity"

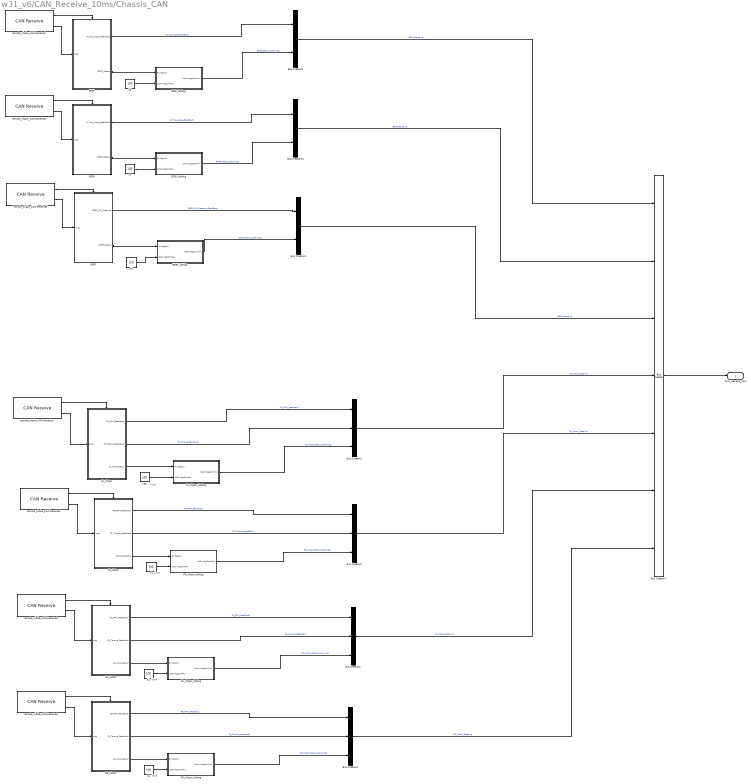
== system w31_v6/CAN_Receive_10ms/Chassis_CAN ==
  note: time
  note: time
  note: time
  note: time
  Bus Creator10 : BusCreator  Inputs=2
  Bus Creator{2..5} (4 alike) : BusCreator  Inputs=3
  Bus Creator6 : BusCreator  Inputs=2
  Bus Creator7 : BusCreator  Inputs=7
  Bus Creator9 : BusCreator  Inputs=2
  DBSF : Subsystem
  DBSF_NoMsg : Subsystem
  EPSF : Subsystem
  EPSF_NoMsg : Subsystem
  EPSR : Subsystem
  EPSR_NoMsg : Subsystem
  FL_Motor : Subsystem
  FL_Motor_NoMsg : Subsystem
  FR_Motor : Subsystem
  FR_Motor_NoMsg : Subsystem
  RL_Motor : Subsystem
  RL_Motor_NoMsg : Subsystem
  RR_Motor : Subsystem
  RR_Motor_NoMsg : Subsystem
  remote_shake_CAN Receive1 : cansrvlib/CAN Receive  useModule=CAN1  messageID=hex2dec('10')  messageType=Standard (11-bit identifier)  t=-1  dataType=CAN_MESSAGE_TYPE  msg_priority=255  messageID_Numeric=16  ECU=V11P51_00E170701_01
  remote_shake_CAN Receive2 : cansrvlib/CAN Receive  useModule=CAN1  messageID=hex2dec('20')  messageType=Standard (11-bit identifier)  t=-1  dataType=CAN_MESSAGE_TYPE  msg_priority=255  messageID_Numeric=32  ECU=V11P51_00E170701_01
  remote_shake_CAN Receive3 : cansrvlib/CAN Receive  useModule=CAN1  messageID=hex2dec('30')  messageType=Standard (11-bit identifier)  t=-1  dataType=CAN_MESSAGE_TYPE  msg_priority=255  messageID_Numeric=48  ECU=V11P51_00E170701_01
  remote_shake_CAN Receive4 : cansrvlib/CAN Receive  useModule=CAN1  messageID=hex2dec('40')  messageType=Standard (11-bit identifier)  t=-1  dataType=CAN_MESSAGE_TYPE  msg_priority=255  messageID_Numeric=64  ECU=V11P51_00E170701_01
  remote_shake_CAN Receive6 : cansrvlib/CAN Receive  useModule=CAN1  messageID=hex2dec('142')  messageType=Standard (11-bit identifier)  t=-1  dataType=CAN_MESSAGE_TYPE  msg_priority=255  messageID_Numeric=322  ECU=V11P51_00E170701_01
  remote_shake_CAN Receive7 : cansrvlib/CAN Receive  useModule=CAN1  messageID=hex2dec('401')  messageType=Standard (11-bit identifier)  t=-1  dataType=CAN_MESSAGE_TYPE  msg_priority=255  messageID_Numeric=1025  ECU=V11P51_00E170701_01
  remote_shake_CAN Receive8 : cansrvlib/CAN Receive  useModule=CAN1  messageID=hex2dec('111')  messageType=Standard (11-bit identifier)  t=-1  dataType=CAN_MESSAGE_TYPE  msg_priority=255  messageID_Numeric=273  ECU=V11P51_00E170701_01
  t{1..3,5..7,10} (7 alike) : Constant  Value=100  OutDataTypeStr=single  SampleTime=-1
  CAN_Receive_Two : Outport
  wires:
  Bus Creator7/1 -> CAN_Receive_Two/1
  EPSF/1(F_Tire_Angle_Feedback) -> Bus Creator9/1  "F_Tire_Angle_Feedback"
  EPSF_NoMsg/1(NoRxMsgComfirm) -> Bus Creator9/2  "EPSF_Status_NoRxMsg"
  EPSR_NoMsg/1(NoRxMsgComfirm) -> Bus Creator10/2  "EPSR_Status_NoRxMsg"
  EPSR/1(R_Tire_Angle_Feedback) -> Bus Creator10/1  "R_Tire_Angle_Feedback"
  remote_shake_CAN Receive1/1 -> FL_Motor/Trigger
  remote_shake_CAN Receive1/2 -> FL_Motor/1(msg)
  FL_Motor/3(FL_MotorStatus) -> FL_Motor_NoMsg/1(RxMsgCnt)
  t10/1 -> FL_Motor_NoMsg/2(NoRxMsgCntMax)
  remote_shake_CAN Receive2/1 -> FR_Motor/Trigger
  remote_shake_CAN Receive2/2 -> FR_Motor/1(msg)
  FR_Motor/3(FR_MotorStatus) -> FR_Motor_NoMsg/1(RxMsgCnt)
  t1/1 -> FR_Motor_NoMsg/2(NoRxMsgCntMax)
  remote_shake_CAN Receive3/1 -> RL_Motor/Trigger
  remote_shake_CAN Receive3/2 -> RL_Motor/1(msg)
  RL_Motor/3(RL_MotorStatus) -> RL_Motor_NoMsg/1(RxMsgCnt)
  t2/1 -> RL_Motor_NoMsg/2(NoRxMsgCntMax)
  remote_shake_CAN Receive4/1 -> RR_Motor/Trigger
  remote_shake_CAN Receive4/2 -> RR_Motor/1(msg)
  RR_Motor/3(RL_MotorStatus) -> RR_Motor_NoMsg/1(RxMsgCnt)
  t3/1 -> RR_Motor_NoMsg/2(NoRxMsgCntMax)
  remote_shake_CAN Receive6/1 -> DBSF/Trigger
  remote_shake_CAN Receive6/2 -> DBSF/1(msg)
  t5/1 -> DBSF_NoMsg/2(NoRxMsgCntMax)
  DBSF/2(DBSF_Status) -> DBSF_NoMsg/1(RxMsgCnt)
  DBSF/1(DBSF_HP_Pressure) -> Bus Creator6/1  "DBSF_HP_Pressure_Feedback"
  DBSF_NoMsg/1(NoRxMsgComfirm) -> Bus Creator6/2  "DBSF_Status_NoRxMsg"
  Bus Creator6/1 -> Bus Creator7/3  "DBSF_Receive"
  Bus Creator9/1 -> Bus Creator7/1  "EPSF_Receive"
  Bus Creator10/1 -> Bus Creator7/2  "EPSR_Receive"
  remote_shake_CAN Receive7/1 -> EPSF/Trigger
  remote_shake_CAN Receive7/2 -> EPSF/1(msg)
  t6/1 -> EPSF_NoMsg/2(NoRxMsgCntMax)
  EPSF/2(EPSF_Status) -> EPSF_NoMsg/1(RxMsgCnt)
  remote_shake_CAN Receive8/1 -> EPSR/Trigger
  remote_shake_CAN Receive8/2 -> EPSR/1(msg)
  t7/1 -> EPSR_NoMsg/2(NoRxMsgCntMax)
  EPSR/2(EPSR_Status) -> EPSR_NoMsg/1(RxMsgCnt)
  Bus Creator2/1 -> Bus Creator7/4  "FL_Motor_Receive"
  Bus Creator3/1 -> Bus Creator7/5  "FR_Motor_Receive"
  Bus Creator4/1 -> Bus Creator7/6  "RL_Motor_Receive"
  Bus Creator5/1 -> Bus Creator7/7  "RR_Motor_Receive"
  FL_Motor/1(FL_RPM_Feedback) -> Bus Creator2/1  "FL_RPM_Feedback"
  FL_Motor/2(FL_Torque_Feedback) -> Bus Creator2/2  "FL_Torque_Feedback"
  FL_Motor_NoMsg/1(NoRxMsgComfirm) -> Bus Creator2/3  "FL_Motor_Status_NoRxMsg"
  FR_Motor/1(FR_RPM_Feedback) -> Bus Creator3/1  "FR_RPM_Feedback"
  FR_Motor/2(FR_Torque_Feedback) -> Bus Creator3/2  "FR_Torque_Feedback"
  FR_Motor_NoMsg/1(NoRxMsgComfirm) -> Bus Creator3/3  "FR_Motor_Status_NoRxMsg"
  RL_Motor/1(RL_RPM_Feedback) -> Bus Creator4/1  "RL_RPM_Feedback"
  RL_Motor/2(RL_Torque_Feedback) -> Bus Creator4/2  "RL_Torque_Feedback"
  RL_Motor_NoMsg/1(NoRxMsgComfirm) -> Bus Creator4/3  "RL_Motor_Status_NoRxMsg"
  RR_Motor/1(RR_RPM_Feedback) -> Bus Creator5/1  "RR_RPM_Feedback"
  RR_Motor/2(FL_Torque_Feedback) -> Bus Creator5/2  "FL_Torque_Feedback"
  RR_Motor_NoMsg/1(NoRxMsgComfirm) -> Bus Creator5/3  "RR_Motor_Status_NoRxMsg"

== system w31_v6/CAN_Receive_10ms/Hardware_Input ==
  Bus Creator18 : BusCreator
  Bus Selector3 : BusSelector  OutputSignals=Key_Ignation,Emergency_Stop,Front_Touch_Switch,Rear_Touch_Switch
  DI signal jittered : Subsystem
  Hardware : Subsystem
  Hardware_Receive : Outport
  wires:
  Hardware/1(Hardware_input) -> Bus Selector3/1
  Bus Selector3/2 -> DI signal jittered/2(Emergency_Stop)  "<Emergency_Stop>"
  Bus Selector3/1 -> DI signal jittered/1(Key_Ignation)  "<Key_Ignation>"
  Bus Creator18/1 -> Hardware_Receive/1  "Hardware_Input"
  DI signal jittered/1(Key_In_Cmd) -> Bus Creator18/1  "Key_Ig_Cmd"
  DI signal jittered/2(Eme_Stop_Cmd) -> Bus Creator18/2  "Eme_Stop_Cmd"
  Bus Selector3/3 -> DI signal jittered/3(Front_Touch_Switch)  "<Front_Touch_Switch>"
  Bus Selector3/4 -> DI signal jittered/4(Rear_Touch_Switch)  "<Rear_Touch_Switch>"
  DI signal jittered/3(Front_Touch_Enable) -> Bus Creator18/3  "Front_Touch_Switch"
  DI signal jittered/4(Rear_Touch_Enable) -> Bus Creator18/4  "Rear_Touch_Switch"

== system w31_v6/CAN_Receive_10ms/Remote_Control_CAN ==
  note: 0-80kph
  note: 0-8Mpa
  note: -30度-+30度
  note: time
  note: time
  Bus Creator : BusCreator  Inputs=2
  Bus Creator1 : BusCreator
  Bus Creator2 : BusCreator  Inputs=9
  Remote_IO_situation1 : Subsystem
  remote_IO_CAN Receive1 : cansrvlib/CAN Receive  useModule=CAN1  messageID=hex2dec('10A')  messageType=Standard (11-bit identifier)  t=-1  dataType=CAN_MESSAGE_TYPE  msg_priority=255  messageID_Numeric=266  ECU=V11P51_00E170701_01
  remote_IO_Stutas1 : Subsystem
  remote_shake1 : Subsystem
  remote_shake_CAN Receive1 : cansrvlib/CAN Receive  useModule=CAN1  messageID=hex2dec('10B')  messageType=Standard (11-bit identifier)  t=-1  dataType=CAN_MESSAGE_TYPE  msg_priority=255  messageID_Numeric=267  ECU=V11P51_00E170701_01
  shake_situation1 : Subsystem
  t10 : Constant  Value=100  OutDataTypeStr=single  SampleTime=-1
  t2 : Constant  Value=100  OutDataTypeStr=single  SampleTime=-1
  Remote_Outside_Control_CAN : Outport
  wires:
  Bus Creator/1 -> Remote_Outside_Control_CAN/1
  remote_shake1/1(Remote_Power_Required) -> Bus Creator1/1  "Remote_Power_Required"
  remote_shake1/3(Remote_Steering_Angle_Required) -> Bus Creator1/3  "Remote_Steering_Angle_Required"
  Bus Creator1/1 -> Bus Creator/1  "Remote_Analog"
  Bus Creator2/1 -> Bus Creator/2  "Remote_IO"
  remote_shake1/2(Remote_Brake_Pressure_Required) -> Bus Creator1/2  "Remote_Brake_Pressure_Required"
  remote_shake_CAN Receive1/1 -> remote_shake1/Trigger
  remote_shake_CAN Receive1/2 -> remote_shake1/1(msg)
  remote_shake1/4(Remote_stutas) -> shake_situation1/1(RxMsgCnt)
  t10/1 -> shake_situation1/2(NoRxMsgCntMax)
  shake_situation1/1(NoRxMsgComfirm) -> Bus Creator1/4  "Remote_Analog_Status"
  remote_IO_CAN Receive1/1 -> remote_IO_Stutas1/Trigger
  remote_IO_CAN Receive1/2 -> remote_IO_Stutas1/1(msg)
  remote_IO_Stutas1/9(Remote_IO_stutas) -> Remote_IO_situation1/1(RxMsgCnt)
  t2/1 -> Remote_IO_situation1/2(NoRxMsgCntMax)
  remote_IO_Stutas1/1(Remote_Control_Speed_or_Torque) -> Bus Creator2/1  "Remote_Control_Speed_or_Torque"
  remote_IO_Stutas1/2(Remote_or_iECU_Mode_Switch) -> Bus Creator2/2  "Remote_or_iECU_Mode_Switch"
  remote_IO_Stutas1/3(Remote_Coordinate_System_Switch) -> Bus Creator2/3  "Remote_Coordinate_System_Switch"
  remote_IO_Stutas1/4(Remote_Steering_Mode_Switch2) -> Bus Creator2/4  "Remote_Steering_Mode_Switch2"
  remote_IO_Stutas1/5(Remote_Gear1) -> Bus Creator2/5  "Remote_Gear1"
  remote_IO_Stutas1/6(EPB_Control_Mode) -> Bus Creator2/6  "EPB_Control_Mode"
  remote_IO_Stutas1/7(Remote_Gear2) -> Bus Creator2/7  "Remote_Gear2"
  remote_IO_Stutas1/8(Remote_Steering_Mode_Switch1) -> Bus Creator2/8  "Remote_Steering_Mode_Switch1"
  Remote_IO_situation1/1(NoRxMsgComfirm) -> Bus Creator2/9  "Remote_IO_Status"

== system w31_v6/CAN_Receive_10ms/Sensor_CAN ==
  Bus Creator1 : BusCreator  Inputs=3
  Bus Creator17 : BusCreator  Inputs=2
  Bus Creator18 : BusCreator  Inputs=2
  Constant1 : Constant  Value=0.5  OutDataTypeStr=single  SampleTime=-1
  Constant2 : Constant  Value=0.5  OutDataTypeStr=single  SampleTime=-1
  Constant3 : Constant  Value=0  OutDataTypeStr=single  SampleTime=-1
  Constant4 : Constant  Value=2  OutDataTypeStr=single  SampleTime=-1
  Constant5 : Constant  Value=0  OutDataTypeStr=single  SampleTime=-1
  CAN_Receive_Inside : Outport
  wires:
  Bus Creator18/1 -> CAN_Receive_Inside/1
  Bus Creator17/1 -> Bus Creator18/1  "IMU_AX_Receive"
  Constant2/1 -> Bus Creator17/1  "Ax"
  Constant3/1 -> Bus Creator17/2  "Ax_NoRxMsg"
  Constant1/1 -> Bus Creator1/1  "Ay"
  Constant5/1 -> Bus Creator1/3  "yaw_ay_NoRxMsg"
  Constant4/1 -> Bus Creator1/2  "yaw"
  Bus Creator1/1 -> Bus Creator18/2  "YAW_AY_Rceive"

== system w31_v6/CAN_Receive_10ms/Status_Cal ==
  Remote : Inport
  Chassis : Inport  Port=2
  iECU : Inport  Port=3
  Hardware : Inport  Port=4
  Subsystem : Subsystem
  Subsystem1 : Subsystem
  Vehicle_Diagnosis : Outport
  Vehicle_Status : Outport  Port=2
  wires:
  Remote/1 -> Subsystem/1(Remote)
  Chassis/1 -> Subsystem/2(Chassis), Subsystem1/2(Chassis)
  Subsystem/1(Vehicle_State) -> Vehicle_Diagnosis/1
  iECU/1 -> Subsystem/3(iECU)
  Hardware/1 -> Subsystem/4(Hardware), Subsystem1/3(Hardware)
  Subsystem/2(Vehicle_Ready) -> Subsystem1/1(Vehicle_Ready)
  Subsystem1/1(Vehicle_Status) -> Vehicle_Status/1

== system w31_v6/CAN_Receive_10ms/iECU_CAN ==
  note: 0-80kph
  note: 0-8Mpa
  note: -30度-+30度
  note: time
  note: -30度-+30度
  Bus Creator1 : BusCreator  Inputs=8
  Constant1 : Constant  Value=0  OutDataTypeStr=Inherit: Inherit via back propagation  SampleTime=-1
  Ground : Ground
  Terminator : Terminator
  iECU : Subsystem
  remote_shake_CAN Receive1 : cansrvlib/CAN Receive  useModule=CAN1  messageID=hex2dec('10C')  messageType=Standard (11-bit identifier)  t=-1  dataType=CAN_MESSAGE_TYPE  msg_priority=255  messageID_Numeric=268  ECU=V11P51_00E170701_01
  shake_situation1 : Subsystem
  t10 : Constant  Value=100  OutDataTypeStr=single  SampleTime=-1
  iECU_CAN : Outport
  wires:
  remote_shake_CAN Receive1/1 -> iECU/Trigger
  remote_shake_CAN Receive1/2 -> iECU/1(msg)
  iECU/7(iECU_Stutas) -> shake_situation1/1(RxMsgCnt)
  t10/1 -> shake_situation1/2(NoRxMsgCntMax)
  Bus Creator1/1 -> iECU_CAN/1
  Ground/1 -> Bus Creator1/4  "iECU_EPB_Req"
  Constant1/1 -> Terminator/1  "iECU_SteeringAngleCmd"
  iECU/1(iECU_Brake_Pressure_Required) -> Bus Creator1/1  "iECU_Brake_Pressure_Required"
  iECU/2(iECU_Control_Flag) -> Bus Creator1/2  "iECU_Control_Flag"
  iECU/3(iECU_Gear_Required) -> Bus Creator1/3  "iECU_Gear_Required"
  iECU/4(iECU_FTire_Angle_Required) -> Bus Creator1/5  "iECU_FTire_Angle_Rrquired"
  iECU/5(iECU_RTire_Angle_Required) -> Bus Creator1/6  "iECU_RTire_Angle_Rrquired"
  iECU/6(iECU_Speed_Required) -> Bus Creator1/7  "iECU_Speed_Required"
  shake_situation1/1(NoRxMsgComfirm) -> Bus Creator1/8  "iECU_Status"
